simulink model "steering_motor_smith"  (R2018b)
settings: Solver=VariableStepAuto  StartTime=0.0  StopTime=10.0  RelTol=1e-3
values from neighbouring files (symbols this model uses):
  D_steering_position = 0.0    (= 0)    [configuration.m]
  delay_tf_steering = 0    [configuration.m]
  den_tf_steering = [1 245.9 0]    [configuration.m]
  den_tf_steering_dis = [den_tf_steering_dis 0] - [0 den_tf_steering_dis]    [configuration.m]
  I_steering_position = 1    [configuration.m]    (also in simulate_bike.m = 30)
  initial_states = [deg2rad(-2) deg2rad(0) deg2rad(0)]    [configuration.m]    (also in configuration_pidTuning.m)
  max_steering_motor_speed = 0.9    [configuration.m]    (also in configuration_pidTuning.m = 7.5)
  min_steering_motor_speed = -0.9    [configuration.m]    (also in configuration_pidTuning.m = -7.5)
  num_tf_steering = [253.4]    [configuration.m]
  num_tf_steering_dis = [num_tf_steering_dis 0]    [configuration.m]
  P_steering_position = 10    [configuration.m]    (also in simulate_bike.m = 30)
  smith_steering = 0    [configuration.m]
  Ts = 0.01    [configuration.m]    (also in configuration_pidTuning.m = 0.04)
libraries: simulink x1
settings Model: Creator=maximef  LastModifiedBy=maximef

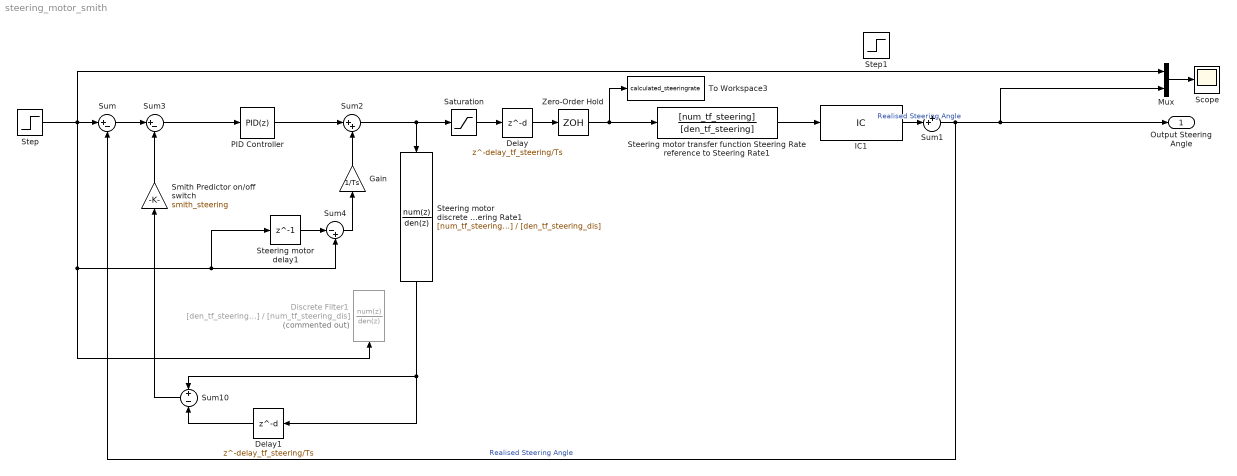
== system steering_motor_smith ==
  Delay : Delay  DelayLength=delay_tf_steering/Ts  SampleTime=Ts
  Delay1 : Delay  DelayLength=delay_tf_steering/Ts  SampleTime=Ts
  Discrete Filter1 : DiscreteFilter  Commented=on  Numerator=[den_tf_steering_dis]  Denominator=[num_tf_steering_dis]
  Gain : Gain  Gain=1/Ts
  IC1 : InitialCondition  Value=initial_states(2)
  Mux : Mux  Inputs=2
  PID Controller : simulink/Continuous/PID Controller  Controller=PID  Form=Parallel  TimeDomain=Discrete-time  SampleTime=Ts  IntegratorMethod=Forward Euler  FilterMethod=Forward Euler  ControllerParametersSource=internal  P=P_steering_position  I=I_steering_position  D=D_steering_position  UseFilter=off  N=1  TunerSelectOption=Transfer Function Based (PID Tuner App)  InitialConditionSource=internal  InitialConditionForIntegrator=0  InitialConditionForFilter=0  DifferentiatorICPrevScaledInput=0  ExternalReset=none  TrackingMode=off  Kt=1  LimitOutput=off  UpperSaturationLimit=inf  LowerSaturationLimit=-inf  LinearizeAsGain=on  AntiWindupMode=none  Kb=1  POutMin=[]  POutMax=[]  IOutMin=[]  IOutMax=[]  DOutMin=[]  DOutMax=[]  NOutMin=[]  NOutMax=[]  SumOutMin=[]  SumOutMax=[]  SaturationOutMin=[]  SaturationOutMax=[]  PParamMin=[]  PParamMax=[]  IParamMin=[]  IParamMax=[]  DParamMin=[]  DParamMax=[]  NParamMin=[]  NParamMax=[]  KbParamMin=[]  KbParamMax=[]  KtParamMin=[]  KtParamMax=[]  KbOutMin=[]  KbOutMax=[]  KtOutMin=[]  KtOutMax=[]  IntegratorOutMin=[]  IntegratorOutMax=[]  FilterOutMin=[]  FilterOutMax=[]  SumI1OutMin=[]  SumI1OutMax=[]  SumI2OutMin=[]  SumI2OutMax=[]  SumI3OutMin=[]  SumI3OutMax=[]  SumI4OutMin=[]  SumI4OutMax=[]  SumDOutMin=[]  SumDOutMax=[]  DifferentiatorOutMin=[]  DifferentiatorOutMax=[]  FilterDiffOutCoefMin=[]  FilterDiffOutCoefMax=[]  ReciprocalOutMin=[]  ReciprocalOutMax=[]  SumDenOutMin=[]  SumDenOutMax=[]  SumNumOutMin=[]  SumNumOutMax=[]  DivideOutMin=[]  DivideOutMax=[]  IntegratorContinuousStateAttributes=''  IntegratorStateMustResolveToSignalObject=off  IntegratorRTWStateStorageClass=Auto  FilterContinuousStateAttributes=''  FilterStateMustResolveToSignalObject=off  FilterRTWStateStorageClass=Auto  ParallelPVariant=InternalParameters  IdealPVariant=Disabled  IVariant=InternalParameters  DVariant=InternalParameters  IntegratorVariant=Discrete  SatVariant=Disabled  AWVariant=Passthrough  PCopyVariant=Disabled  TRVariant=Disabled  FdbkBlocksVariant=Forward  IdealPFdbkVariant=Disabled  SatFdbkVariant=Disabled  DerivativeFilterVariant=Differentiator  NVariant=Passthrough  NCopyVariant=Disabled_SignalSpec  FilterICVariant=InternalICsDifferentiator  IntegratorICVariant=InternalICs  ExternalResetVariant=Disabled  TRSumVariant=Passthrough  SumFdbkVariant=Disabled  SumVariant=Sum_PID
  Saturation : Saturate  UpperLimit=max_steering_motor_speed  LowerLimit=min_steering_motor_speed
  Scope : Scope
  Smith Predictor on/off switch : Gain  Gain=smith_steering
  Steering motor delay1 : Delay  DelayLength=1  SampleTime=Ts
  Steering motor discrete transfer function Steering Rate reference to Steering Rate1 : DiscreteTransferFcn  Numerator=[num_tf_steering_dis]  Denominator=[den_tf_steering_dis]  SampleTime=Ts
  Steering motor transfer function Steering Rate reference to Steering Rate1 : TransferFcn  Numerator=[num_tf_steering]  Denominator=[den_tf_steering]
  Step : Step  Time=5  After=deg2rad(3)  SampleTime=0
  Step1 : Step  Time=3  After=deg2rad(2)  SampleTime=0
  Sum : Sum  Inputs=|+-
  Sum1 : Sum  Inputs=++|
  Sum10 : Sum  Inputs=+-
  Sum2 : Sum  Inputs=|++
  Sum3 : Sum  Inputs=|+-
  Sum4 : Sum  Inputs=|-+
  To Workspace3 : ToWorkspace  VariableName=calculated_steeringrate  SaveFormat=Timeseries  SampleTime=-1
  Zero-Order Hold : ZeroOrderHold  SampleTime=Ts
  Output Steering Angle : Outport
  wires:
  Delay/1 -> Zero-Order Hold/1
  Sum1/1 -> Sum/2, Output Steering Angle/1, Mux/2  "Realised Steering Angle"
  Sum/1 -> Sum3/1
  Steering motor transfer function Steering Rate reference to Steering Rate1/1 -> IC1/1
  Smith Predictor on/off switch/1 -> Sum3/2
  Step/1 -> Steering motor delay1/1, Sum4/2, Discrete Filter1/1, Sum/1, Mux/1
  Sum3/1 -> PID Controller/1
  Delay1/1 -> Sum10/2
  Sum10/1 -> Smith Predictor on/off switch/1
  Mux/1 -> Scope/1
  Sum2/1 -> Saturation/1, Steering motor discrete transfer function Steering Rate reference to Steering Rate1/1
  Steering motor discrete transfer function Steering Rate reference to Steering Rate1/1 -> Delay1/1, Sum10/1
  PID Controller/1 -> Sum2/1
  Saturation/1 -> Delay/1
  Zero-Order Hold/1 -> Steering motor transfer function Steering Rate reference to Steering Rate1/1, To Workspace3/1
  IC1/1 -> Sum1/2  "Realised Steering Angle"
  Sum4/1 -> Gain/1
  Steering motor delay1/1 -> Sum4/1
  Gain/1 -> Sum2/2
